simulink model "ofdm_pktdetector_mimo"  (Simulink 6.6)
settings: Solver=ode45  StartTime=0.0  StopTime=simTime  RelTol=1e-3
PreLoadFcn:
  | init
PostLoadFcn:
  | init
InitFcn:
  | init
StartFcn:
  | init
undefined symbols (not defined in the file or in its folder): gcbh, xlBlockLoadCallback, xlGetSimulinkPeriod
libraries: xbsIndex_r4 x201
(part 2 of 3)

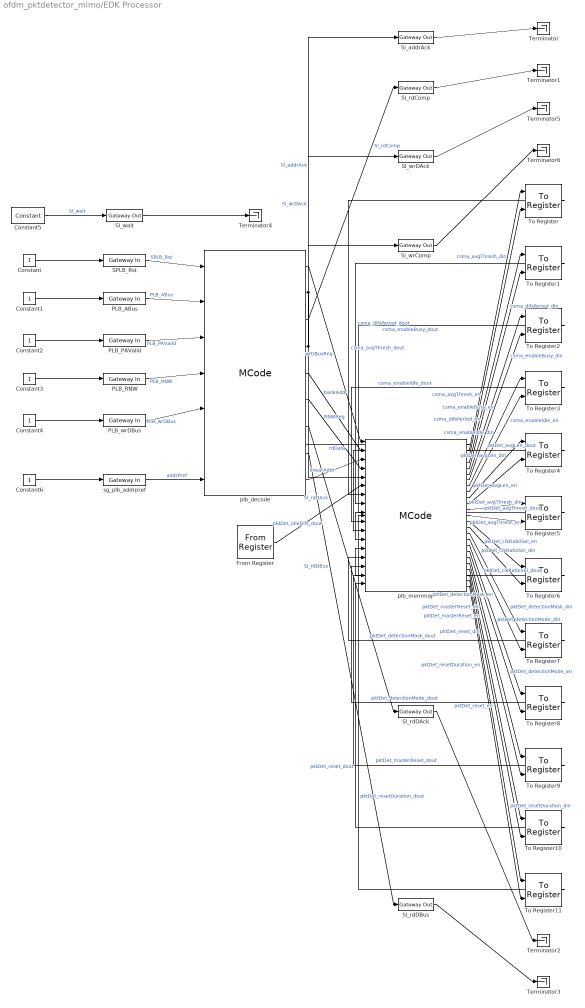
== system ofdm_pktdetector_mimo/EDK Processor ==
  Constant{,1..4,6} (6 alike) : Constant
  Constant5 : xbsIndex_r4/Constant  arith_type=Unsigned  const=0  n_bits=1  bin_pt=0  explicit_period=on  period=xlGetSimulinkPeriod(gcb)  equ=P=C  opselect=C  inp2=PCIN>>17  opr=+  inp1=P  carry=CIN  dbl_ovrd=off  block_type=constant
      settings: block_version=10.1.2
  From Register : xbsIndex_r4/From Register  shared_memory_name='pktDet_idleDifs'  init=0  period=xlGetSimulinkPeriod(gcb)  ownership=Owned and initialized elsewhere  arith_type=Unsigned  n_bits=1  bin_pt=0  dbl_ovrd=off  block_type=fromreg
      settings: AttributesFormatString=<< %<shared_memory_name> >>  infoedit="Register block that reads data to a shared memory register.  Delay of one sample period."  block_version=10.1.2
  PLB_ABus : xbsIndex_r4/Gateway In  arith_type=Unsigned  n_bits=32  bin_pt=0  quantization="Round  (unbiased: +/- Inf)"  overflow=Saturate  period=xlGetSimulinkPeriod(gcb)  dbl_ovrd=off  timing_constraint=None  locs_specified=off  LOCs={}  block_type=gatewayin
      settings: infoedit="Gateway in block.  Converts inputs of type Simulink integer, double and fixed point to  Xilinx fixed point type.<P><P>Hardware notes:  In hardware these blocks become top level input ports."  sginterface={'Xilinx'=>{'jtaghwcosim'=>{'non_memory_mapped_port'=>'PLB_ABus'}},'iopad'=>{'constraint'=>'#'}}  block_version=10.1.2
  PLB_PAValid : xbsIndex_r4/Gateway In  arith_type=Unsigned  n_bits=1  bin_pt=0  quantization="Round  (unbiased: +/- Inf)"  overflow=Saturate  period=xlGetSimulinkPeriod(gcb)  dbl_ovrd=off  timing_constraint=None  locs_specified=off  LOCs={}  block_type=gatewayin
      settings: infoedit="Gateway in block.  Converts inputs of type Simulink integer, double and fixed point to  Xilinx fixed point type.<P><P>Hardware notes:  In hardware these blocks become top level input ports."  sginterface={'Xilinx'=>{'jtaghwcosim'=>{'non_memory_mapped_port'=>'PLB_PAValid'}},'iopad'=>{'constraint'=>'#'}}  block_version=10.1.2
  PLB_RNW : xbsIndex_r4/Gateway In  arith_type=Unsigned  n_bits=1  bin_pt=0  quantization="Round  (unbiased: +/- Inf)"  overflow=Saturate  period=xlGetSimulinkPeriod(gcb)  dbl_ovrd=off  timing_constraint=None  locs_specified=off  LOCs={}  block_type=gatewayin
      settings: infoedit="Gateway in block.  Converts inputs of type Simulink integer, double and fixed point to  Xilinx fixed point type.<P><P>Hardware notes:  In hardware these blocks become top level input ports."  sginterface={'Xilinx'=>{'jtaghwcosim'=>{'non_memory_mapped_port'=>'PLB_RNW'}},'iopad'=>{'constraint'=>'#'}}  block_version=10.1.2
  PLB_wrDBus : xbsIndex_r4/Gateway In  arith_type=Unsigned  n_bits=32  bin_pt=0  quantization="Round  (unbiased: +/- Inf)"  overflow=Saturate  period=xlGetSimulinkPeriod(gcb)  dbl_ovrd=off  timing_constraint=None  locs_specified=off  LOCs={}  block_type=gatewayin
      settings: infoedit="Gateway in block.  Converts inputs of type Simulink integer, double and fixed point to  Xilinx fixed point type.<P><P>Hardware notes:  In hardware these blocks become top level input ports."  sginterface={'Xilinx'=>{'jtaghwcosim'=>{'non_memory_mapped_port'=>'PLB_wrDBus'}},'iopad'=>{'constraint'=>'#'}}  block_version=10.1.2
  SPLB_Rst : xbsIndex_r4/Gateway In  arith_type=Unsigned  n_bits=1  bin_pt=0  quantization="Round  (unbiased: +/- Inf)"  overflow=Saturate  period=xlGetSimulinkPeriod(gcb)  dbl_ovrd=off  timing_constraint=None  locs_specified=off  LOCs={}  block_type=gatewayin
      settings: infoedit="Gateway in block.  Converts inputs of type Simulink integer, double and fixed point to  Xilinx fixed point type.<P><P>Hardware notes:  In hardware these blocks become top level input ports."  sginterface={'Xilinx'=>{'jtaghwcosim'=>{'non_memory_mapped_port'=>'SPLB_Rst'}},'iopad'=>{'constraint'=>'#'}}  block_version=10.1.2
  Sl_addrAck : xbsIndex_r4/Gateway Out  hdl_port=on  timing_constraint=None  locs_specified=off  LOCs={}  block_type=gatewayout
      settings: infoedit="Gateway out block.  Converts Xilinx fixed point inputs into ouputs of type Simulink integer, double, or fixed point.<P><P>Hardware notes:  In hardware these blocks become top level output ports or are discarded, depending on how they are configured."  sginterface={'Xilinx'=>{'jtaghwcosim'=>{'non_memory_mapped_port'=>'Sl_addrAck'}},'iopad'=>{'constraint'=>'#'}}  block_version=10.1.2
  Sl_rdComp : xbsIndex_r4/Gateway Out  hdl_port=on  timing_constraint=None  locs_specified=off  LOCs={}  block_type=gatewayout
      settings: infoedit="Gateway out block.  Converts Xilinx fixed point inputs into ouputs of type Simulink integer, double, or fixed point.<P><P>Hardware notes:  In hardware these blocks become top level output ports or are discarded, depending on how they are configured."  sginterface={'Xilinx'=>{'jtaghwcosim'=>{'non_memory_mapped_port'=>'Sl_rdComp'}},'iopad'=>{'constraint'=>'#'}}  block_version=10.1.2
  Sl_rdDAck : xbsIndex_r4/Gateway Out  hdl_port=on  timing_constraint=None  locs_specified=off  LOCs={}  block_type=gatewayout
      settings: infoedit="Gateway out block.  Converts Xilinx fixed point inputs into ouputs of type Simulink integer, double, or fixed point.<P><P>Hardware notes:  In hardware these blocks become top level output ports or are discarded, depending on how they are configured."  sginterface={'Xilinx'=>{'jtaghwcosim'=>{'non_memory_mapped_port'=>'Sl_rdDAck'}},'iopad'=>{'constraint'=>'#'}}  block_version=10.1.2
  Sl_rdDBus : xbsIndex_r4/Gateway Out  hdl_port=on  timing_constraint=None  locs_specified=off  LOCs={}  block_type=gatewayout
      settings: infoedit="Gateway out block.  Converts Xilinx fixed point inputs into ouputs of type Simulink integer, double, or fixed point.<P><P>Hardware notes:  In hardware these blocks become top level output ports or are discarded, depending on how they are configured."  sginterface={'Xilinx'=>{'jtaghwcosim'=>{'non_memory_mapped_port'=>'Sl_rdDBus'}},'iopad'=>{'constraint'=>'#'}}  block_version=10.1.2
  Sl_wait : xbsIndex_r4/Gateway Out  hdl_port=on  timing_constraint=None  locs_specified=off  LOCs={}  block_type=gatewayout
      settings: infoedit="Gateway out block.  Converts Xilinx fixed point inputs into ouputs of type Simulink integer, double, or fixed point.<P><P>Hardware notes:  In hardware these blocks become top level output ports or are discarded, depending on how they are configured."  sginterface={'Xilinx'=>{'jtaghwcosim'=>{'non_memory_mapped_port'=>'Sl_wait'}},'iopad'=>{'constraint'=>'#'}}  block_version=10.1.2
  Sl_wrComp : xbsIndex_r4/Gateway Out  hdl_port=on  timing_constraint=None  locs_specified=off  LOCs={}  block_type=gatewayout
      settings: infoedit="Gateway out block.  Converts Xilinx fixed point inputs into ouputs of type Simulink integer, double, or fixed point.<P><P>Hardware notes:  In hardware these blocks become top level output ports or are discarded, depending on how they are configured."  sginterface={'Xilinx'=>{'jtaghwcosim'=>{'non_memory_mapped_port'=>'Sl_wrComp'}},'iopad'=>{'constraint'=>'#'}}  block_version=10.1.2
  Sl_wrDAck : xbsIndex_r4/Gateway Out  hdl_port=on  timing_constraint=None  locs_specified=off  LOCs={}  block_type=gatewayout
      settings: infoedit="Gateway out block.  Converts Xilinx fixed point inputs into ouputs of type Simulink integer, double, or fixed point.<P><P>Hardware notes:  In hardware these blocks become top level output ports or are discarded, depending on how they are configured."  sginterface={'Xilinx'=>{'jtaghwcosim'=>{'non_memory_mapped_port'=>'Sl_wrDAck'}},'iopad'=>{'constraint'=>'#'}}  block_version=10.1.2
  Terminator{,1..6} (7 alike) : Terminator
  To Register : xbsIndex_r4/To Register  shared_memory_name='csma_avgThresh'  init=0  ownership=Owned and initialized elsewhere  explicit_data_type=on  arith_type=Unsigned  n_bits=16  bin_pt=0  dbl_ovrd=off  block_type=toreg
      settings: AttributesFormatString=<< %<shared_memory_name> >>  infoedit="Register block that writes data to a shared memory register.  Delay of one sample period."  block_version=10.1.2
  To Register1 : xbsIndex_r4/To Register  shared_memory_name='csma_difsPeriod'  init=0  ownership=Owned and initialized elsewhere  explicit_data_type=on  arith_type=Unsigned  n_bits=10  bin_pt=0  dbl_ovrd=off  block_type=toreg
      settings: AttributesFormatString=<< %<shared_memory_name> >>  infoedit="Register block that writes data to a shared memory register.  Delay of one sample period."  block_version=10.1.2
  To Register10 : xbsIndex_r4/To Register  shared_memory_name='pktDet_reset'  init=0  ownership=Owned and initialized elsewhere  explicit_data_type=on  arith_type=Unsigned  n_bits=1  bin_pt=0  dbl_ovrd=off  block_type=toreg
      settings: AttributesFormatString=<< %<shared_memory_name> >>  infoedit="Register block that writes data to a shared memory register.  Delay of one sample period."  block_version=10.1.2
  To Register11 : xbsIndex_r4/To Register  shared_memory_name='pktDet_resetDuration'  init=0  ownership=Owned and initialized elsewhere  explicit_data_type=on  arith_type=Unsigned  n_bits=16  bin_pt=0  dbl_ovrd=off  block_type=toreg
      settings: AttributesFormatString=<< %<shared_memory_name> >>  infoedit="Register block that writes data to a shared memory register.  Delay of one sample period."  block_version=10.1.2
  To Register2 : xbsIndex_r4/To Register  shared_memory_name='csma_enableBusy'  init=0  ownership=Owned and initialized elsewhere  explicit_data_type=on  arith_type=Unsigned  n_bits=1  bin_pt=0  dbl_ovrd=off  block_type=toreg
      settings: AttributesFormatString=<< %<shared_memory_name> >>  infoedit="Register block that writes data to a shared memory register.  Delay of one sample period."  block_version=10.1.2
  To Register3 : xbsIndex_r4/To Register  shared_memory_name='csma_enableIdle'  init=0  ownership=Owned and initialized elsewhere  explicit_data_type=on  arith_type=Unsigned  n_bits=1  bin_pt=0  dbl_ovrd=off  block_type=toreg
      settings: AttributesFormatString=<< %<shared_memory_name> >>  infoedit="Register block that writes data to a shared memory register.  Delay of one sample period."  block_version=10.1.2
  To Register4 : xbsIndex_r4/To Register  shared_memory_name='pktDet_avgLen'  init=0  ownership=Owned and initialized elsewhere  explicit_data_type=on  arith_type=Unsigned  n_bits=5  bin_pt=0  dbl_ovrd=off  block_type=toreg
      settings: AttributesFormatString=<< %<shared_memory_name> >>  infoedit="Register block that writes data to a shared memory register.  Delay of one sample period."  block_version=10.1.2
  To Register5 : xbsIndex_r4/To Register  shared_memory_name='pktDet_avgThresh'  init=0  ownership=Owned and initialized elsewhere  explicit_data_type=on  arith_type=Unsigned  n_bits=16  bin_pt=0  dbl_ovrd=off  block_type=toreg
      settings: AttributesFormatString=<< %<shared_memory_name> >>  infoedit="Register block that writes data to a shared memory register.  Delay of one sample period."  block_version=10.1.2
  To Register6 : xbsIndex_r4/To Register  shared_memory_name='pktDet_clkRatioSel'  init=0  ownership=Owned and initialized elsewhere  explicit_data_type=on  arith_type=Unsigned  n_bits=1  bin_pt=0  dbl_ovrd=off  block_type=toreg
      settings: AttributesFormatString=<< %<shared_memory_name> >>  infoedit="Register block that writes data to a shared memory register.  Delay of one sample period."  block_version=10.1.2
  To Register7 : xbsIndex_r4/To Register  shared_memory_name='pktDet_detectionMask'  init=0  ownership=Owned and initialized elsewhere  explicit_data_type=on  arith_type=Unsigned  n_bits=4  bin_pt=0  dbl_ovrd=off  block_type=toreg
      settings: AttributesFormatString=<< %<shared_memory_name> >>  infoedit="Register block that writes data to a shared memory register.  Delay of one sample period."  block_version=10.1.2
  To Register8 : xbsIndex_r4/To Register  shared_memory_name='pktDet_detectionMode'  init=0  ownership=Owned and initialized elsewhere  explicit_data_type=on  arith_type=Unsigned  n_bits=1  bin_pt=0  dbl_ovrd=off  block_type=toreg
      settings: AttributesFormatString=<< %<shared_memory_name> >>  infoedit="Register block that writes data to a shared memory register.  Delay of one sample period."  block_version=10.1.2
  To Register9 : xbsIndex_r4/To Register  shared_memory_name='pktDet_masterReset'  init=0  ownership=Owned and initialized elsewhere  explicit_data_type=on  arith_type=Unsigned  n_bits=1  bin_pt=0  dbl_ovrd=off  block_type=toreg
      settings: AttributesFormatString=<< %<shared_memory_name> >>  infoedit="Register block that writes data to a shared memory register.  Delay of one sample period."  block_version=10.1.2
  plb_decode : xbsIndex_r4/MCode  mfname=xlmax  explicit_period=off  period=1  dbl_ovrd=off  enable_stdout=off  enable_debug=off  mfilecontent=|  suppress_output=1  defparams={}  hide_port_list={}  block_type=mcode
      | function [wrDBusReg, addrAck, rdComp, wrDAck, bankAddr, RNWReg, rdDAck, rdDBus, linearAddr] = ...
      |     plb_bus_decode(plbRst, plbABus, plbPAValid, plbRNW, plbWrDBus, rdData, addrPref)
      | 
      | % constant variables (TODO: should pass from outside)
      | ADDRPREF_LEN = 20;
      | BANKADDR_LEN = 2;
      | LINEARADDR_LEN = 8;
      | ABUS_LEN = 32;
      | DBUS_LEN = 32;
      | 
      | % declare and initialize persistent variables
      | % register input bus signals
      | persistent plbRstReg_, plbRstReg_ = xl_state(0, {xlBoolean});
      | persistent plbABusReg_, plbABusReg_ = xl_state(0, {xlUnsigned, ABUS_LEN, 0});
      | persistent plbPAValidReg_, plbPAValidReg_ = xl_state(0, {xlBoolean});
      | persistent plbRNWReg_, plbRNWReg_ = xl_state(0, {xlUnsigned, 1, 0});
      | persistent plbWrDBusReg_, plbWrDBusReg_ = xl_state(0, {xlUnsigned, DBUS_LEN, 0});
      | 
      | % ===== rest of the outputs =====
      | 
      | bankAddr   = xl_slice(plbABusReg_, 2+BANKADDR_LEN+LINEARADDR_LEN-1, 2+LINEARADDR_LEN);
      | linearAddr = xl_slice(plbABusReg_, 2+LINEARADDR_LEN-1, 2);
      | RNWReg = plbRNWReg_;
      | wrDBusReg = plbWrDBusReg_;
      | 
      | % ===== p_select =====
      | 
      | % register PAValid
      | persistent aValidReg, aValidReg = xl_state(0, {xlBoolean});
      | aValidReg = plbPAValidReg_;
      | 
      | % extract and register the address prefix
      | addrPref_in = xl_slice(plbABusReg_, xl_nbits(plbABusReg_)-1, xl_nbits(plbABusReg_)-ADDRPREF_LEN);
      | if addrPref_in == addrPref
      |     ps1 = true;
      | else 
      |     ps1 = false;
      | end 
      | 
      | persistent ps1Reg, ps1Reg = xl_state(0, ps1);
      | ps1Reg = ps1;
      | 
      | ps = xl_and(ps1Reg, aValidReg);
      | 
      | % ===== addrAck =====
      | 
      | % register ps
      | persistent psReg, psReg = xl_state(0, ps);
      | 
      | addrAck = xfix({xlUnsigned, 1, 0}, xl_and(xl_not(plbRstReg_), ps, xl_not(psReg)));
      | 
      | psReg = ps;
      | 
      | % ===== rdComp, rd/wr DAck =====
      |  
      | rdComp1 = xfix({xlUnsigned, 1, 0}, xl_and(addrAck, RNWReg));
      | 
      | NUM_rdCompDelay = 3;
      | persistent rdCompDelay, rdCompDelay = xl_state(zeros(1, NUM_rdCompDelay), rdComp1, NUM_rdCompDelay);
      | rdComp2 = rdCompDelay.back;
      | rdCompDelay.push_front_pop_back(rdComp1);
      | 
      | persistent rdCompReg, rdCompReg = xl_state(0, rdComp1);
      | rdComp = rdCompReg;
      | rdCompReg = rdComp2;
      | 
      | persistent rdDAckReg, rdDAckReg = xl_state(0, rdComp1);
      | rdDAck = rdDAckReg;
      | rdDAckReg = rdComp;
      | 
      | persistent wrDAckReg, wrDAckReg = xl_state(0, addrAck);
      | wrDAck = wrDAckReg;
      | wrDAckReg = xl_and(addrAck, xl_not(RNWReg));
      | 
      | % ===== rdDBus =====
      | 
      | rdSel = xl_or(rdComp2, rdComp);
      | 
      | if rdSel == 1
      |     rdDBus1 = rdData;
      | else
      |     rdDBus1 = 0;
      | end % if
      | 
      | persistent rdDBusReg, rdDBusReg = xl_state(0, rdDBus1);
      | rdDBus = rdDBusReg;
      | rdDBusReg = rdDBus1;
      | 
      | % rdDBus = xl_concat(rdDBus32, rdDBus32);
      | % rdDBus = rdDBus32;
      | 
      | % ===== update the persistent variables =====
      | 
      | plbRstReg_ = plbRst;
      | plbABusReg_ = plbABus;
      | plbPAValidReg_ = plbPAValid;
      | plbRNWReg_ = plbRNW;
      | plbWrDBusReg_ = xl_slice(plbWrDBus, DBUS_LEN-1, 0);
      settings: block_version=10.1.2
  plb_memmap : xbsIndex_r4/MCode  mfname=xlmax  explicit_period=off  period=1  dbl_ovrd=off  enable_stdout=off  enable_debug=off  mfilecontent=|  suppress_output=1  defparams={}  hide_port_list={}  block_type=mcode
      | function [read_bank_out, sm_csma_avgThresh_din, sm_csma_avgThresh_en, sm_csma_difsPeriod_din, sm_csma_difsPeriod_en, sm_csma_enableBusy_din, sm_csma_enableBusy_en, sm_csma_enableIdle_din, sm_csma_enableIdle_en, sm_pktDet_avgLen_din, sm_pktDet_avgLen_en, sm_pktDet_avgThresh_din, sm_pktDet_avgThresh_en, sm_pktDet_clkRatioSel_din, sm_pktDet_clkRatioSel_en, sm_pktDet_detectionMask_din, sm_pktDet_detectionMask_en, sm_pktDet_detectionMode_din, sm_pktDet_detectionMode_en, sm_pktDet_masterReset_din, sm_pktDet_masterReset_en, sm_pktDet_reset_din, sm_pktDet_reset_en, sm_pktDet_resetDuration_din, sm_pktDet_resetDuration_en] = plb_memmap_select(wrDBus, bankAddr, linearAddr, RNWReg, addrAck, sm_pktDet_idleDifs, sm_csma_avgThresh, sm_csma_difsPeriod, sm_csma_enableBusy, sm_csma_enableIdle, sm_pktDet_avgLen, sm_pktDet_avgThresh, sm_pktDet_clkRatioSel, sm_pktDet_detectionMask, sm_pktDet_detectionMode, sm_pktDet_masterReset, sm_pktDet_reset, sm_pktDet_resetDuration)
      | 
      | 
      | % connvert the input data to UFix_32_0 (the bus data type)
      | % 'From Register' blocks
      | % sm_pktDet_idleDifs_bus = xfix({xlUnsigned, 32, 0}, 0);
      | sm_pktDet_idleDifs_bus = xl_force(sm_pktDet_idleDifs, xlUnsigned, 0);
      | 
      | % 'To Register' blocks
      | % sm_csma_avgThresh_dout = xfix({xlUnsigned, 32, 0}, 0);
      | sm_csma_avgThresh_dout = xl_force(sm_csma_avgThresh, xlUnsigned, 0);
      | 
      | % sm_csma_difsPeriod_dout = xfix({xlUnsigned, 32, 0}, 0);
      | sm_csma_difsPeriod_dout = xl_force(sm_csma_difsPeriod, xlUnsigned, 0);
      | 
      | % sm_csma_enableBusy_dout = xfix({xlUnsigned, 32, 0}, 0);
      | sm_csma_enableBusy_dout = xl_force(sm_csma_enableBusy, xlUnsigned, 0);
      | 
      | % sm_csma_enableIdle_dout = xfix({xlUnsigned, 32, 0}, 0);
      | sm_csma_enableIdle_dout = xl_force(sm_csma_enableIdle, xlUnsigned, 0);
      | 
      | % sm_pktDet_avgLen_dout = xfix({xlUnsigned, 32, 0}, 0);
      | sm_pktDet_avgLen_dout = xl_force(sm_pktDet_avgLen, xlUnsigned, 0);
      | 
      | % sm_pktDet_avgThresh_dout = xfix({xlUnsigned, 32, 0}, 0);
      | sm_pktDet_avgThresh_dout = xl_force(sm_pktDet_avgThresh, xlUnsigned, 0);
      | 
      | % sm_pktDet_clkRatioSel_dout = xfix({xlUnsigned, 32, 0}, 0);
      | sm_pktDet_clkRatioSel_dout = xl_force(sm_pktDet_clkRatioSel, xlUnsigned, 0);
      | 
      | % sm_pktDet_detectionMask_dout = xfix({xlUnsigned, 32, 0}, 0);
      | sm_pktDet_detectionMask_dout = xl_force(sm_pktDet_detectionMask, xlUnsigned, 0);
      | 
      | % sm_pktDet_detectionMode_dout = xfix({xlUnsigned, 32, 0}, 0);
      | sm_pktDet_detectionMode_dout = xl_force(sm_pktDet_detectionMode, xlUnsigned, 0);
      | 
      | % sm_pktDet_masterReset_dout = xfix({xlUnsigned, 32, 0}, 0);
      | sm_pktDet_masterReset_dout = xl_force(sm_pktDet_masterReset, xlUnsigned, 0);
      | 
      | % sm_pktDet_reset_dout = xfix({xlUnsigned, 32, 0}, 0);
      | sm_pktDet_reset_dout = xl_force(sm_pktDet_reset, xlUnsigned, 0);
      | 
      | % sm_pktDet_resetDuration_dout = xfix({xlUnsigned, 32, 0}, 0);
      | sm_pktDet_resetDuration_dout = xl_force(sm_pktDet_resetDuration, xlUnsigned, 0);
      | 
      | % 'From FIFO' blocks
      | % 'To FIFO' blocks
      | % 'Shared Memory' blocks
      | 
      | % 'dout' ports of 'From Register' blocks
      | 
      | % registered register mux output
      | persistent reg_bank_out_reg; reg_bank_out_reg = xl_state(0, {xlUnsigned, 32, 0});
      | reg_bank_out = reg_bank_out_reg;
      | 
      | if linearAddr == 12
      |     reg_bank_out_reg = sm_pktDet_idleDifs_bus;
      | elseif linearAddr == 0
      |     reg_bank_out_reg = sm_csma_avgThresh_dout;
      | elseif linearAddr == 1
      |     reg_bank_out_reg = sm_csma_difsPeriod_dout;
      | elseif linearAddr == 2
      |     reg_bank_out_reg = sm_csma_enableBusy_dout;
      | elseif linearAddr == 3
      |     reg_bank_out_reg = sm_csma_enableIdle_dout;
      | elseif linearAddr == 4
      |     reg_bank_out_reg = sm_pktDet_avgLen_dout;
      | elseif linearAddr == 5
      |     reg_bank_out_reg = sm_pktDet_avgThresh_dout;
      | elseif linearAddr == 6
      |     reg_bank_out_reg = sm_pktDet_clkRatioSel_dout;
      | elseif linearAddr == 7
      |     reg_bank_out_reg = sm_pktDet_detectionMask_dout;
      | elseif linearAddr == 8
      |     reg_bank_out_reg = sm_pktDet_detectionMode_dout;
      | elseif linearAddr == 9
      |     reg_bank_out_reg = sm_pktDet_masterReset_dout;
      | elseif linearAddr == 10
      |     reg_bank_out_reg = sm_pktDet_reset_dout;
      | elseif linearAddr == 11
      |     reg_bank_out_reg = sm_pktDet_resetDuration_dout;
      | end
      | 
      | 
      | % 'From FIFO' and 'To FIFO' blocks
      | 
      | 
      | 
      | 
      | 
      | opCode = xl_concat(addrAck, RNWReg, bankAddr, linearAddr);
      | 
      | % 'Shared Memory' blocks
      | 
      | 
      | 
      | 
      | 
      | % 'din' ports of 'Shared Memory' blocks
      | 
      | 
      | % 'we' ports of 'Shared Memory' blocks
      | 
      | 
      | % 'addr' ports of 'Shared Memory' blocks
      | 
      | 
      | % 're' ports of 'From FIFO' blocks
      | 
      | 
      | % 'en' ports of 'To Register' blocks
      | if opCode == xl_concat(xfix({xlUnsigned, 4, 0}, 10), ...
      |                        xfix({xlUnsigned, xl_nbits(linearAddr), 0}, 0))
      |     sm_csma_avgThresh_en = true;
      | else
      |     sm_csma_avgThresh_en = false;
      | end
      | if opCode == xl_concat(xfix({xlUnsigned, 4, 0}, 10), ...
      |                        xfix({xlUnsigned, xl_nbits(linearAddr), 0}, 1))
      |     sm_csma_difsPeriod_en = true;
      | else
      |     sm_csma_difsPeriod_en = false;
      | end
      | if opCode == xl_concat(xfix({xlUnsigned, 4, 0}, 10), ...
      |                        xfix({xlUnsigned, xl_nbits(linearAddr), 0}, 2))
      |     sm_csma_enableBusy_en = true;
      | else
      |     sm_csma_enableBusy_en = false;
      | end
      | if opCode == xl_concat(xfix({xlUnsigned, 4, 0}, 10), ...
      |                        xfix({xlUnsigned, xl_nbits(linearAddr), 0}, 3))
      |     sm_csma_enableIdle_en = true;
      | else
      |     sm_csma_enableIdle_en = false;
      | end
      | if opCode == xl_concat(xfix({xlUnsigned, 4, 0}, 10), ...
      |                        xfix({xlUnsigned, xl_nbits(linearAddr), 0}, 4))
      |     sm_pktDet_avgLen_en = true;
      | else
      |     sm_pktDet_avgLen_en = false;
      | end
      | if opCode == xl_concat(xfix({xlUnsigned, 4, 0}, 10), ...
      |                        xfix({xlUnsigned, xl_nbits(linearAddr), 0}, 5))
      |     sm_pktDet_avgThresh_en = true;
      | else
      |     sm_pktDet_avgThresh_en = false;
      | end
      | if opCode == xl_concat(xfix({xlUnsigned, 4, 0}, 10), ...
      |                        xfix({xlUnsigned, xl_nbits(linearAddr), 0}, 6))
      |     sm_pktDet_clkRatioSel_en = true;
      | else
      |     sm_pktDet_clkRatioSel_en = false;
      | end
      | if opCode == xl_concat(xfix({xlUnsigned, 4, 0}, 10), ...
      |                        xfix({xlUnsigned, xl_nbits(linearAddr), 0}, 7))
      |     sm_pktDet_detectionMask_en = true;
      | else
      |     sm_pktDet_detectionMask_en = false;
      | end
      | if opCode == xl_concat(xfix({xlUnsigned, 4, 0}, 10), ...
      |                        xfix({xlUnsigned, xl_nbits(linearAddr), 0}, 8))
      |     sm_pktDet_detectionMode_en = true;
      | else
      |     sm_pktDet_detectionMode_en = false;
      | end
      | if opCode == xl_concat(xfix({xlUnsigned, 4, 0}, 10), ...
      |                        xfix({xlUnsigned, xl_nbits(linearAddr), 0}, 9))
      |     sm_pktDet_masterReset_en = true;
      | else
      |     sm_pktDet_masterReset_en = false;
      | end
      | if opCode == xl_concat(xfix({xlUnsigned, 4, 0}, 10), ...
      |                        xfix({xlUnsigned, xl_nbits(linearAddr), 0}, 10))
      |     sm_pktDet_reset_en = true;
      | else
      |     sm_pktDet_reset_en = false;
      | end
      | if opCode == xl_concat(xfix({xlUnsigned, 4, 0}, 10), ...
      |                        xfix({xlUnsigned, xl_nbits(linearAddr), 0}, 11))
      |     sm_pktDet_resetDuration_en = true;
      | else
      |     sm_pktDet_resetDuration_en = false;
      | end
      | 
      | 
      | % 'din' ports of 'To FIFO' blocks
      | 
      | 
      | % 'we' ports of 'To FIFO' blocks
      | 
      | 
      | % 'din' ports of 'To Register' blocks
      | sm_csma_avgThresh_din = xl_force(xl_slice(wrDBus, 16 - 1, 0), ...
      |                                  xlUnsigned, ...
      |                                  0);
      | sm_csma_difsPeriod_din = xl_force(xl_slice(wrDBus, 10 - 1, 0), ...
      |                                  xlUnsigned, ...
      |                                  0);
      | sm_csma_enableBusy_din = xl_force(xl_slice(wrDBus, 1 - 1, 0), ...
      |                                  xlUnsigned, ...
      |                                  0);
      | sm_csma_enableIdle_din = xl_force(xl_slice(wrDBus, 1 - 1, 0), ...
      |                                  xlUnsigned, ...
      |                                  0);
      | sm_pktDet_avgLen_din = xl_force(xl_slice(wrDBus, 5 - 1, 0), ...
      |                                  xlUnsigned, ...
      |                                  0);
      | sm_pktDet_avgThresh_din = xl_force(xl_slice(wrDBus, 16 - 1, 0), ...
      |                                  xlUnsigned, ...
      |                                  0);
      | sm_pktDet_clkRatioSel_din = xl_force(xl_slice(wrDBus, 1 - 1, 0), ...
      |                                  xlUnsigned, ...
      |                                  0);
      | sm_pktDet_detectionMask_din = xl_force(xl_slice(wrDBus, 4 - 1, 0), ...
      |                                  xlUnsigned, ...
      |                                  0);
      | sm_pktDet_detectionMode_din = xl_force(xl_slice(wrDBus, 1 - 1, 0), ...
      |                                  xlUnsigned, ...
      |                                  0);
      | sm_pktDet_masterReset_din = xl_force(xl_slice(wrDBus, 1 - 1, 0), ...
      |                                  xlUnsigned, ...
      |                                  0);
      | sm_pktDet_reset_din = xl_force(xl_slice(wrDBus, 1 - 1, 0), ...
      |                                  xlUnsigned, ...
      |                                  0);
      | sm_pktDet_resetDuration_din = xl_force(xl_slice(wrDBus, 16 - 1, 0), ...
      |                                  xlUnsigned, ...
      |                                  0);
      | 
      | 
      | persistent read_bank_out_reg; read_bank_out_reg = xl_state(0, {xlUnsigned, 32, 0});
      | read_bank_out = read_bank_out_reg;
      | 
      | persistent bankAddr_reg; bankAddr_reg = xl_state(0, bankAddr);
      | 
      | if bankAddr_reg == 0
      |     % Bank 0: Shared Memories
      |     read_bank_out_reg = 0;
      | elseif bankAddr_reg == 1
      |     % Bank 1: From/To FIFOs
      |     read_bank_out_reg =  0;
      | elseif bankAddr_reg == 2
      |     % Bank 1: From/To Registers
      |     read_bank_out_reg = reg_bank_out;
      | elseif bankAddr_reg == 3
      |     % Bank 1: Configure Registers
      |     read_bank_out_reg = 0;
      | end
      | 
      | bankAddr_reg = bankAddr;
      settings: block_version=10.1.2
  sg_plb_addrpref : xbsIndex_r4/Gateway In  arith_type=Unsigned  n_bits=20  bin_pt=0  quantization="Round  (unbiased: +/- Inf)"  overflow=Saturate  period=xlGetSimulinkPeriod(gcb)  dbl_ovrd=off  timing_constraint=None  locs_specified=off  LOCs={}  block_type=gatewayin
      settings: infoedit="Gateway in block.  Converts inputs of type Simulink integer, double and fixed point to  Xilinx fixed point type.<P><P>Hardware notes:  In hardware these blocks become top level input ports."  sginterface={'Xilinx'=>{'jtaghwcosim'=>{'non_memory_mapped_port'=>'sg_plb_addrpref'}},'iopad'=>{'constraint'=>'#'}}  block_version=10.1.2
  wires:
  plb_decode/2 -> plb_memmap/5, Sl_addrAck/1  "Sl_addrAck"
  plb_decode/4 -> Sl_wrDAck/1, Sl_wrComp/1  "Sl_wrDAck"
  plb_memmap/25 -> To Register11/2  "pktDet_resetDuration_en"
  plb_memmap/24 -> To Register11/1  "pktDet_resetDuration_din"
  plb_memmap/23 -> To Register10/2  "pktDet_reset_en"
  plb_memmap/22 -> To Register10/1  "pktDet_reset_din"
  plb_memmap/21 -> To Register9/2  "pktDet_masterReset_en"
  plb_memmap/20 -> To Register9/1  "pktDet_masterReset_din"
  plb_memmap/19 -> To Register8/2  "pktDet_detectionMode_en"
  plb_memmap/18 -> To Register8/1  "pktDet_detectionMode_din"
  plb_memmap/17 -> To Register7/2  "pktDet_detectionMask_en"
  plb_memmap/16 -> To Register7/1  "pktDet_detectionMask_din"
  plb_memmap/15 -> To Register6/2  "pktDet_clkRatioSel_en"
  plb_memmap/14 -> To Register6/1  "pktDet_clkRatioSel_din"
  plb_memmap/13 -> To Register5/2  "pktDet_avgThresh_en"
  plb_memmap/12 -> To Register5/1  "pktDet_avgThresh_din"
  plb_memmap/11 -> To Register4/2  "pktDet_avgLen_en"
  plb_memmap/10 -> To Register4/1  "pktDet_avgLen_din"
  plb_memmap/9 -> To Register3/2  "csma_enableIdle_en"
  plb_memmap/8 -> To Register3/1  "csma_enableIdle_din"
  plb_memmap/7 -> To Register2/2  "csma_enableBusy_en"
  plb_memmap/6 -> To Register2/1  "csma_enableBusy_din"
  plb_memmap/5 -> To Register1/2  "csma_difsPeriod_en"
  plb_memmap/4 -> To Register1/1  "csma_difsPeriod_din"
  plb_memmap/3 -> To Register/2  "csma_avgThresh_en"
  plb_memmap/2 -> To Register/1  "csma_avgThresh_din"
  plb_memmap/1 -> plb_decode/6  "rdData"
  To Register11/1 -> plb_memmap/18  "pktDet_resetDuration_dout"
  To Register10/1 -> plb_memmap/17  "pktDet_reset_dout"
  To Register9/1 -> plb_memmap/16  "pktDet_masterReset_dout"
  To Register8/1 -> plb_memmap/15  "pktDet_detectionMode_dout"
  To Register7/1 -> plb_memmap/14  "pktDet_detectionMask_dout"
  To Register6/1 -> plb_memmap/13  "pktDet_clkRatioSel_dout"
  To Register5/1 -> plb_memmap/12  "pktDet_avgThresh_dout"
  To Register4/1 -> plb_memmap/11  "pktDet_avgLen_dout"
  To Register3/1 -> plb_memmap/10  "csma_enableIdle_dout"
  To Register2/1 -> plb_memmap/9  "csma_enableBusy_dout"
  To Register1/1 -> plb_memmap/8  "csma_difsPeriod_dout"
  To Register/1 -> plb_memmap/7  "csma_avgThresh_dout"
  From Register/1 -> plb_memmap/6  "pktDet_idleDifs_dout"
  plb_decode/6 -> plb_memmap/4  "RNWReg"
  plb_decode/9 -> plb_memmap/3  "linearAddr"
  plb_decode/5 -> plb_memmap/2  "bankAddr"
  plb_decode/1 -> plb_memmap/1  "wrDBusReg"
  plb_decode/8 -> Sl_rdDBus/1  "Sl_rdDBus"
  plb_decode/7 -> Sl_rdDAck/1  "Sl_rdDAck"
  plb_decode/3 -> Sl_rdComp/1  "Sl_rdComp"
  sg_plb_addrpref/1 -> plb_decode/7  "addrPref"
  PLB_wrDBus/1 -> plb_decode/5  "PLB_wrDBus"
  PLB_RNW/1 -> plb_decode/4  "PLB_RNW"
  PLB_PAValid/1 -> plb_decode/3  "PLB_PAValid"
  PLB_ABus/1 -> plb_decode/2  "PLB_ABus"
  SPLB_Rst/1 -> plb_decode/1  "SPLB_Rst"
  Constant6/1 -> sg_plb_addrpref/1
  Constant5/1 -> Sl_wait/1  "Sl_wait"
  Constant4/1 -> PLB_wrDBus/1
  Constant3/1 -> PLB_RNW/1
  Constant2/1 -> PLB_PAValid/1
  Constant1/1 -> PLB_ABus/1
  Constant/1 -> SPLB_Rst/1
  Sl_wrComp/1 -> Terminator6/1
  Sl_wrDAck/1 -> Terminator5/1
  Sl_wait/1 -> Terminator4/1
  Sl_rdDBus/1 -> Terminator3/1
  Sl_rdDAck/1 -> Terminator2/1
  Sl_rdComp/1 -> Terminator1/1
  Sl_addrAck/1 -> Terminator/1

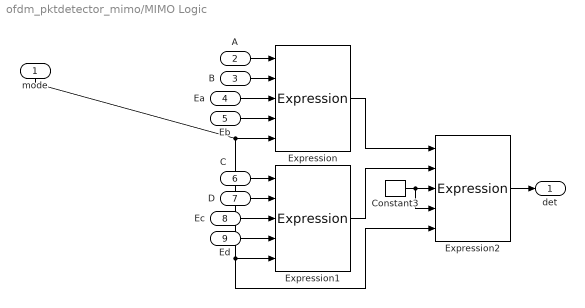
== system ofdm_pktdetector_mimo/MIMO Logic ==
  mode : Inport  Orientation=down
  A : Inport  Port=2
  B : Inport  Port=3
  Ea : Inport  Port=4
  Eb : Inport  Port=5
  C : Inport  Port=6
  D : Inport  Port=7
  Ec : Inport  Port=8
  Ed : Inport  Port=9
  Constant3 : xbsIndex_r4/Constant  arith_type=Unsigned  const=1  n_bits=1  bin_pt=0  explicit_period=off  period=1  equ=P=C  opselect=C  inp2=PCIN>>17  opr=+  inp1=P  carry=CIN  dbl_ovrd=off  block_type=constant
      settings: block_version=8.2
  Expression : xbsIndex_r4/Expression  expression=(~M&~Ea&Eb&~A&B)|(~M&~Ea&Eb&A&B)|(~M&Ea&~Eb&A&~Eb)|(~M&Ea&~Eb&A&B)|(~M&Ea&Eb&A&B)|(M&~Ea&Eb&~A&B)|(M&~Ea&Eb&A&B)|(M&Ea&~Eb&A&~B)|(M&Ea&~Eb&A&B)|(M&Ea&Eb&~A&B)|(M&Ea&Eb&A&~B)|(M&Ea&Eb&A&B)  align_bp=on  en=off  latency=0  precision=Full  arith_type=Unsigned  n_bits=16  bin_pt=0  dbl_ovrd=off  block_type=expr
      settings: block_version=8.2
  Expression1 : xbsIndex_r4/Expression  expression=(~M&~Ea&Eb&~A&B)|(~M&~Ea&Eb&A&B)|(~M&Ea&~Eb&A&~Eb)|(~M&Ea&~Eb&A&B)|(~M&Ea&Eb&A&B)|(M&~Ea&Eb&~A&B)|(M&~Ea&Eb&A&B)|(M&Ea&~Eb&A&~B)|(M&Ea&~Eb&A&B)|(M&Ea&Eb&~A&B)|(M&Ea&Eb&A&~B)|(M&Ea&Eb&A&B)  align_bp=on  en=off  latency=0  precision=Full  arith_type=Unsigned  n_bits=16  bin_pt=0  dbl_ovrd=off  block_type=expr
      settings: block_version=8.2
  Expression2 : xbsIndex_r4/Expression  expression=(~M&~Ea&Eb&~A&B)|(~M&~Ea&Eb&A&B)|(~M&Ea&~Eb&A&~Eb)|(~M&Ea&~Eb&A&B)|(~M&Ea&Eb&A&B)|(M&~Ea&Eb&~A&B)|(M&~Ea&Eb&A&B)|(M&Ea&~Eb&A&~B)|(M&Ea&~Eb&A&B)|(M&Ea&Eb&~A&B)|(M&Ea&Eb&A&~B)|(M&Ea&Eb&A&B)  align_bp=on  en=off  latency=0  precision=Full  arith_type=Unsigned  n_bits=16  bin_pt=0  dbl_ovrd=off  block_type=expr
      settings: block_version=8.2
  det : Outport
  wires:
  mode/1 -> Expression2/5, Expression1/5, Expression/5
  Constant3/1 -> Expression2/3, Expression2/4
  Expression1/1 -> Expression2/2
  Expression/1 -> Expression2/1
  Ea/1 -> Expression/3
  Eb/1 -> Expression/4
  Ec/1 -> Expression1/3
  Ed/1 -> Expression1/4
  A/1 -> Expression/1
  B/1 -> Expression/2
  C/1 -> Expression1/1
  Expression2/1 -> det/1
  D/1 -> Expression1/2

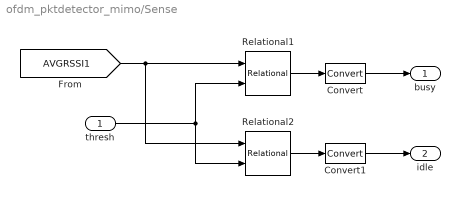
== system ofdm_pktdetector_mimo/Sense ==
  thresh : Inport
  Convert : xbsIndex_r4/Convert  arith_type=Unsigned  n_bits=1  bin_pt=0  quantization=Truncate  overflow=Wrap  latency=0  dbl_ovrd=off  pipeline=off  block_type=convert
      settings: block_version=8.2
  Convert1 : xbsIndex_r4/Convert  arith_type=Unsigned  n_bits=1  bin_pt=0  quantization=Truncate  overflow=Wrap  latency=0  dbl_ovrd=off  pipeline=off  block_type=convert
      settings: block_version=8.2
  Relational1 : xbsIndex_r4/Relational  mode=a>b  en=off  latency=0  dbl_ovrd=off  block_type=relational
      settings: block_version=VER_STRING_GOES_HERE
  Relational2 : xbsIndex_r4/Relational  mode=a<b  en=off  latency=0  dbl_ovrd=off  block_type=relational
      settings: block_version=VER_STRING_GOES_HERE
  busy : Outport
  idle : Outport  Port=2
  wires:
  [AVGRSSI1] -> Relational1/1, Relational2/1
  thresh/1 -> Relational2/2, Relational1/2
  Relational1/1 -> Convert/1
  Relational2/1 -> Convert1/1
  Convert/1 -> busy/1
  Convert1/1 -> idle/1

== system ofdm_pktdetector_mimo/Sense1 ==
  thresh : Inport
  Convert : xbsIndex_r4/Convert  arith_type=Unsigned  n_bits=1  bin_pt=0  quantization=Truncate  overflow=Wrap  latency=0  dbl_ovrd=off  pipeline=off  block_type=convert
      settings: block_version=8.2
  Convert1 : xbsIndex_r4/Convert  arith_type=Unsigned  n_bits=1  bin_pt=0  quantization=Truncate  overflow=Wrap  latency=0  dbl_ovrd=off  pipeline=off  block_type=convert
      settings: block_version=8.2
  Relational1 : xbsIndex_r4/Relational  mode=a>b  en=off  latency=0  dbl_ovrd=off  block_type=relational
      settings: block_version=VER_STRING_GOES_HERE
  Relational2 : xbsIndex_r4/Relational  mode=a<b  en=off  latency=0  dbl_ovrd=off  block_type=relational
      settings: block_version=VER_STRING_GOES_HERE
  busy : Outport
  idle : Outport  Port=2
  wires:
  Convert1/1 -> idle/1
  Convert/1 -> busy/1
  Relational2/1 -> Convert1/1
  Relational1/1 -> Convert/1
  thresh/1 -> Relational1/2, Relational2/2
  [AVGRSSI2] -> Relational2/1, Relational1/1

== system ofdm_pktdetector_mimo/Sense2 ==
  thresh : Inport
  Convert : xbsIndex_r4/Convert  arith_type=Unsigned  n_bits=1  bin_pt=0  quantization=Truncate  overflow=Wrap  latency=0  dbl_ovrd=off  pipeline=off  block_type=convert
      settings: block_version=8.2
  Convert1 : xbsIndex_r4/Convert  arith_type=Unsigned  n_bits=1  bin_pt=0  quantization=Truncate  overflow=Wrap  latency=0  dbl_ovrd=off  pipeline=off  block_type=convert
      settings: block_version=8.2
  Relational1 : xbsIndex_r4/Relational  mode=a>b  en=off  latency=0  dbl_ovrd=off  block_type=relational
      settings: block_version=VER_STRING_GOES_HERE
  Relational2 : xbsIndex_r4/Relational  mode=a<b  en=off  latency=0  dbl_ovrd=off  block_type=relational
      settings: block_version=VER_STRING_GOES_HERE
  busy : Outport
  idle : Outport  Port=2
  wires:
  [AVGRSSI3] -> Relational1/1, Relational2/1
  thresh/1 -> Relational2/2, Relational1/2
  Relational1/1 -> Convert/1
  Relational2/1 -> Convert1/1
  Convert/1 -> busy/1
  Convert1/1 -> idle/1

== system ofdm_pktdetector_mimo/Sense3 ==
  thresh : Inport
  Convert : xbsIndex_r4/Convert  arith_type=Unsigned  n_bits=1  bin_pt=0  quantization=Truncate  overflow=Wrap  latency=0  dbl_ovrd=off  pipeline=off  block_type=convert
      settings: block_version=8.2
  Convert1 : xbsIndex_r4/Convert  arith_type=Unsigned  n_bits=1  bin_pt=0  quantization=Truncate  overflow=Wrap  latency=0  dbl_ovrd=off  pipeline=off  block_type=convert
      settings: block_version=8.2
  Relational1 : xbsIndex_r4/Relational  mode=a>b  en=off  latency=0  dbl_ovrd=off  block_type=relational
      settings: block_version=VER_STRING_GOES_HERE
  Relational2 : xbsIndex_r4/Relational  mode=a<b  en=off  latency=0  dbl_ovrd=off  block_type=relational
      settings: block_version=VER_STRING_GOES_HERE
  busy : Outport
  idle : Outport  Port=2
  wires:
  Convert1/1 -> idle/1
  Convert/1 -> busy/1
  Relational2/1 -> Convert1/1
  Relational1/1 -> Convert/1
  thresh/1 -> Relational1/2, Relational2/2
  [AVGRSSI4] -> Relational2/1, Relational1/1

== system ofdm_pktdetector_mimo/Detection1/averager ==
  raw : Inport
  reset : Inport  Port=2
  avglen : Inport  Port=3
  Accumulator : xbsIndex_r4/Accumulator  operation=Add  n_bits=16  overflow=Flag as error  scale=1  rst=on  hasbypass=off  en=off  dbl_ovrd=off  use_behavioral_HDL=on  block_type=accum
      settings: infoedit="Adder or subtractor-based accumulator.   Output type and binary point position match the input.<P><P>Hardware notes: When \"Reinitialize with input 'b' on reset\" is selected, the accumulator is forced to run at the system rate even if the input 'b' is running at a slower rate."  block_version=VER_STRING_GOES_HERE
  AddSub : xbsIndex_r4/AddSub  mode=Subtraction  use_carryin=off  use_carryout=off  en=off  latency=0  precision=Full  arith_type=Unsigned  n_bits=10  bin_pt=0  quantization=Truncate  overflow=Wrap  dbl_ovrd=off  use_behavioral_HDL=off  pipelined=off  use_rpm=on  block_type=addsub
      settings: block_version=VER_STRING_GOES_HERE
  Addressable Shift Register : xbsIndex_r4/Addressable Shift Register  infer_latency=on  depth=2  initVector=[0]  en=off  dbl_ovrd=off  use_behavioral_HDL=off  use_rpm=off  block_type=addrsr
      settings: infoedit="Delay of  configurable length.  Any element  in the delay     line   can    be   addressed   and   driven    onto   the   output     port.<P><P>Hardware  notes: Implemented  using SRL16s.     If Virtex-4, Virtex-II or Spartan-3 devices are used, multiple SRLC16s are cascaded together."  block_version=VER_STRING_GOES_HERE
  Register : xbsIndex_r4/Register  init=0  rst=on  en=off  dbl_ovrd=off  block_type=register
      settings: block_version=VER_STRING_GOES_HERE
  avg : Outport
  wires:
  Addressable Shift Register/1 -> AddSub/2
  AddSub/1 -> Accumulator/1
  Register/1 -> Addressable Shift Register/1, AddSub/1
  avglen/1 -> Addressable Shift Register/2
  raw/1 -> Register/1
  Accumulator/1 -> avg/1
  reset/1 -> Register/2, Accumulator/2

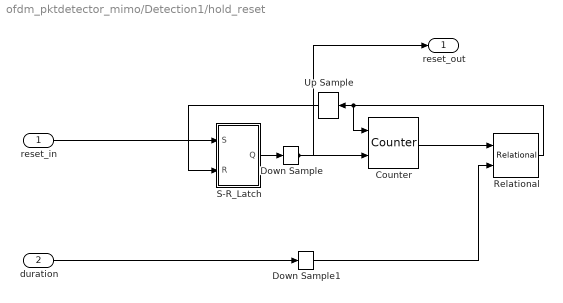
== system ofdm_pktdetector_mimo/Detection1/hold_reset ==
  reset_in : Inport
  duration : Inport  Port=2
  Counter : xbsIndex_r4/Counter  cnt_type=Free Running  cnt_to=0  operation=Up  start_count=0  cnt_by_val=1  arith_type=Unsigned  n_bits=8  bin_pt=0  load_pin=off  rst=on  en=on  explicit_period=on  period=1  dbl_ovrd=off  use_behavioral_HDL=off  use_rpm=off  block_type=counter
      settings: block_version=VER_STRING_GOES_HERE
  Down Sample : xbsIndex_r4/Down Sample  sample_ratio=4  sample_phase="Last Value of Frame  (most efficient)"  en=off  latency=1  dbl_ovrd=off  block_type=dsamp
      settings: block_version=VER_STRING_GOES_HERE
  Down Sample1 : xbsIndex_r4/Down Sample  sample_ratio=4  sample_phase="Last Value of Frame  (most efficient)"  en=off  latency=1  dbl_ovrd=off  block_type=dsamp
      settings: block_version=VER_STRING_GOES_HERE
  Relational : xbsIndex_r4/Relational  mode=a=b  en=off  latency=0  dbl_ovrd=off  block_type=relational
      settings: block_version=VER_STRING_GOES_HERE
  S-R_Latch : Subsystem
  Up Sample : xbsIndex_r4/Up Sample  Orientation=left  sample_ratio=4  copy_samples=on  dbl_ovrd=off  block_type=usamp
      settings: infoedit="Up samples input data.  Inserted values  can be zeros or copies of the most recent input sample.<P><P>Hardware notes: No hardware is needed if inserted values are copies of the input sample; otherwise, a mux and single bit flip-flop are used."  block_version=VER_STRING_GOES_HERE
  reset_out : Outport
  wires:
  Relational/1 -> Counter/1, Up Sample/1
  S-R_Latch/1(Q) -> Down Sample/1
  Counter/1 -> Relational/1
  reset_in/1 -> S-R_Latch/1(S)
  duration/1 -> Down Sample1/1
  Down Sample/1 -> Counter/2, reset_out/1
  Down Sample1/1 -> Relational/2
  Up Sample/1 -> S-R_Latch/2(R)

== system ofdm_pktdetector_mimo/Detection1/posedge3 ==
  In : Inport
  Delay : xbsIndex_r4/Delay  en=off  latency=1  dbl_ovrd=off  reg_retiming=off  block_type=delay
      settings: infoedit=Hardware notes: A delay line is a chain, each link of which is an SRL16 followed by a flip-flop. If register retiming is enabled, the delay line is a chain of flip-flops.  xl_area=[1 1 0 0 0 0 0]  block_version=8.2
  Inverter : xbsIndex_r4/Inverter  en=off  latency=0  dbl_ovrd=off  block_type=inv
      settings: xl_area=[0 0 0 0 0 0 0]  block_version=8.2
  Logical : xbsIndex_r4/Logical  logical_function=AND  inputs=2  en=off  latency=0  precision=Full  arith_type=Unsigned  n_bits=16  bin_pt=0  align_bp=on  dbl_ovrd=off  block_type=logical
      settings: xl_area=[1 0 0 1 0 0 0]  block_version=8.2
  Out : Outport
  wires:
  Delay/1 -> Inverter/1
  Inverter/1 -> Logical/2
  In/1 -> Logical/1, Delay/1
  Logical/1 -> Out/1

== system ofdm_pktdetector_mimo/Detection2/averager ==
  raw : Inport
  reset : Inport  Port=2
  avglen : Inport  Port=3
  Accumulator : xbsIndex_r4/Accumulator  operation=Add  n_bits=16  overflow=Flag as error  scale=1  rst=on  hasbypass=off  en=off  dbl_ovrd=off  use_behavioral_HDL=on  block_type=accum
      settings: infoedit="Adder or subtractor-based accumulator.   Output type and binary point position match the input.<P><P>Hardware notes: When \"Reinitialize with input 'b' on reset\" is selected, the accumulator is forced to run at the system rate even if the input 'b' is running at a slower rate."  block_version=VER_STRING_GOES_HERE
  AddSub : xbsIndex_r4/AddSub  mode=Subtraction  use_carryin=off  use_carryout=off  en=off  latency=0  precision=Full  arith_type=Unsigned  n_bits=10  bin_pt=0  quantization=Truncate  overflow=Wrap  dbl_ovrd=off  use_behavioral_HDL=off  pipelined=off  use_rpm=on  block_type=addsub
      settings: block_version=VER_STRING_GOES_HERE
  Addressable Shift Register : xbsIndex_r4/Addressable Shift Register  infer_latency=on  depth=2  initVector=[0]  en=off  dbl_ovrd=off  use_behavioral_HDL=off  use_rpm=off  block_type=addrsr
      settings: infoedit="Delay of  configurable length.  Any element  in the delay     line   can    be   addressed   and   driven    onto   the   output     port.<P><P>Hardware  notes: Implemented  using SRL16s.     If Virtex-4, Virtex-II or Spartan-3 devices are used, multiple SRLC16s are cascaded together."  block_version=VER_STRING_GOES_HERE
  Register : xbsIndex_r4/Register  init=0  rst=on  en=off  dbl_ovrd=off  block_type=register
      settings: block_version=VER_STRING_GOES_HERE
  avg : Outport
  wires:
  reset/1 -> Accumulator/2, Register/2
  Accumulator/1 -> avg/1
  raw/1 -> Register/1
  avglen/1 -> Addressable Shift Register/2
  Register/1 -> AddSub/1, Addressable Shift Register/1
  AddSub/1 -> Accumulator/1
  Addressable Shift Register/1 -> AddSub/2

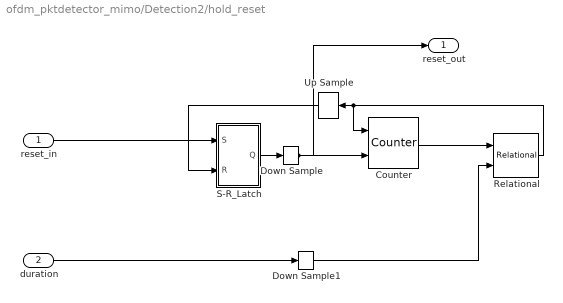
== system ofdm_pktdetector_mimo/Detection2/hold_reset ==
  reset_in : Inport
  duration : Inport  Port=2
  Counter : xbsIndex_r4/Counter  cnt_type=Free Running  cnt_to=0  operation=Up  start_count=0  cnt_by_val=1  arith_type=Unsigned  n_bits=8  bin_pt=0  load_pin=off  rst=on  en=on  explicit_period=on  period=1  dbl_ovrd=off  use_behavioral_HDL=off  use_rpm=off  block_type=counter
      settings: block_version=VER_STRING_GOES_HERE
  Down Sample : xbsIndex_r4/Down Sample  sample_ratio=4  sample_phase="Last Value of Frame  (most efficient)"  en=off  latency=1  dbl_ovrd=off  block_type=dsamp
      settings: block_version=VER_STRING_GOES_HERE
  Down Sample1 : xbsIndex_r4/Down Sample  sample_ratio=4  sample_phase="Last Value of Frame  (most efficient)"  en=off  latency=1  dbl_ovrd=off  block_type=dsamp
      settings: block_version=VER_STRING_GOES_HERE
  Relational : xbsIndex_r4/Relational  mode=a=b  en=off  latency=0  dbl_ovrd=off  block_type=relational
      settings: block_version=VER_STRING_GOES_HERE
  S-R_Latch : Subsystem
  Up Sample : xbsIndex_r4/Up Sample  Orientation=left  sample_ratio=4  copy_samples=on  dbl_ovrd=off  block_type=usamp
      settings: infoedit="Up samples input data.  Inserted values  can be zeros or copies of the most recent input sample.<P><P>Hardware notes: No hardware is needed if inserted values are copies of the input sample; otherwise, a mux and single bit flip-flop are used."  block_version=VER_STRING_GOES_HERE
  reset_out : Outport
  wires:
  Up Sample/1 -> S-R_Latch/2(R)
  Down Sample1/1 -> Relational/2
  Down Sample/1 -> reset_out/1, Counter/2
  duration/1 -> Down Sample1/1
  reset_in/1 -> S-R_Latch/1(S)
  Counter/1 -> Relational/1
  S-R_Latch/1(Q) -> Down Sample/1
  Relational/1 -> Up Sample/1, Counter/1

== system ofdm_pktdetector_mimo/Detection2/posedge3 ==
  In : Inport
  Delay : xbsIndex_r4/Delay  en=off  latency=1  dbl_ovrd=off  reg_retiming=off  block_type=delay
      settings: infoedit=Hardware notes: A delay line is a chain, each link of which is an SRL16 followed by a flip-flop. If register retiming is enabled, the delay line is a chain of flip-flops.  xl_area=[1 1 0 0 0 0 0]  block_version=8.2
  Inverter : xbsIndex_r4/Inverter  en=off  latency=0  dbl_ovrd=off  block_type=inv
      settings: xl_area=[0 0 0 0 0 0 0]  block_version=8.2
  Logical : xbsIndex_r4/Logical  logical_function=AND  inputs=2  en=off  latency=0  precision=Full  arith_type=Unsigned  n_bits=16  bin_pt=0  align_bp=on  dbl_ovrd=off  block_type=logical
      settings: xl_area=[1 0 0 1 0 0 0]  block_version=8.2
  Out : Outport
  wires:
  Logical/1 -> Out/1
  In/1 -> Delay/1, Logical/1
  Inverter/1 -> Logical/2
  Delay/1 -> Inverter/1

== system ofdm_pktdetector_mimo/Detection3/averager ==
  raw : Inport
  reset : Inport  Port=2
  avglen : Inport  Port=3
  Accumulator : xbsIndex_r4/Accumulator  operation=Add  n_bits=16  overflow=Flag as error  scale=1  rst=on  hasbypass=off  en=off  dbl_ovrd=off  use_behavioral_HDL=on  block_type=accum
      settings: infoedit="Adder or subtractor-based accumulator.   Output type and binary point position match the input.<P><P>Hardware notes: When \"Reinitialize with input 'b' on reset\" is selected, the accumulator is forced to run at the system rate even if the input 'b' is running at a slower rate."  block_version=VER_STRING_GOES_HERE
  AddSub : xbsIndex_r4/AddSub  mode=Subtraction  use_carryin=off  use_carryout=off  en=off  latency=0  precision=Full  arith_type=Unsigned  n_bits=10  bin_pt=0  quantization=Truncate  overflow=Wrap  dbl_ovrd=off  use_behavioral_HDL=off  pipelined=off  use_rpm=on  block_type=addsub
      settings: block_version=VER_STRING_GOES_HERE
  Addressable Shift Register : xbsIndex_r4/Addressable Shift Register  infer_latency=on  depth=2  initVector=[0]  en=off  dbl_ovrd=off  use_behavioral_HDL=off  use_rpm=off  block_type=addrsr
      settings: infoedit="Delay of  configurable length.  Any element  in the delay     line   can    be   addressed   and   driven    onto   the   output     port.<P><P>Hardware  notes: Implemented  using SRL16s.     If Virtex-4, Virtex-II or Spartan-3 devices are used, multiple SRLC16s are cascaded together."  block_version=VER_STRING_GOES_HERE
  Register : xbsIndex_r4/Register  init=0  rst=on  en=off  dbl_ovrd=off  block_type=register
      settings: block_version=VER_STRING_GOES_HERE
  avg : Outport
  wires:
  Addressable Shift Register/1 -> AddSub/2
  AddSub/1 -> Accumulator/1
  Register/1 -> Addressable Shift Register/1, AddSub/1
  avglen/1 -> Addressable Shift Register/2
  raw/1 -> Register/1
  Accumulator/1 -> avg/1
  reset/1 -> Register/2, Accumulator/2
